simulink model "rti1401_program_controls_2018_test"  (R2017b)
settings: Solver=ode1  StartTime=0.0  StopTime=Inf  FixedStep=0.001  RelTol=1e-3  EnableMultiTasking=on
PreLoadFcn:
  | dataCar
  | load_vars
  | structAero
  | structEstimPar
  | structSensors
  | structSettings
PostLoadFcn:
  | , if any(exist('dsrtsu_mdlpostloadfcn', 'file') == [2, 3, 6]), try dsrtsu_mdlpostloadfcn('Execute', bdroot); catch fprintf('Error in PostLoadFcn (dsrtsu_mdlpostloadfcn) for model "%s":\n %s\n', bdroot, lasterr); end, end,
InitFcn:
  | dataCar
  | load_vars
  | structAero
  | structEstimPar
  | structSensors
  | structSettings
StartFcn:
  | dataCar
  | load_vars
  | structAero
  | structEstimPar
  | structSensors
  | structSettings
values from neighbouring files (symbols this model uses):
  Throttle_limits = [0.15, 0.90, 0.16, 0.92]    [load_vars.m]
undefined symbols (not defined in the file or in its folder): car, sensors
libraries: rtican x44, hdlsllib x32, simulink x8, rti1401lib_II_base x1
(part 1 of 11)
settings Model: DSRTSU_INTERNAL_RTI_VER=490  DSRTSU_INTERNAL_RTI_TYPE=rti1401  DSRTSU_INTERNAL_RTIFPGA=80  DSRTSU_INTERNAL_MDBS_VER=10  Creator=Arthur Coppieters  LastModifiedBy=User
settings OptimizationCC: BlockReduction=off  OptimizeBlockIOStorage=off  BufferReuse=off  GlobalBufferReuse=off  ExpressionFolding=off  LocalBlockOutputs=off  LifeSpan=inf
settings DebuggingCC: SFUnexpectedBacktrackingDiag=warning  SFNoUnconditionalDefaultTransitionDiag=warning  SFExecutionAtInitializationDiag=none
settings HardwareCC: ProdBitPerPointer=32  ProdBitPerSizeT=32  ProdBitPerPtrDiffT=32  ProdLargestAtomicInteger=Integer  ProdEndianess=BigEndian  ProdWordSize=32  ProdHWDeviceType=Custom Processor->Custom  TargetIntDivRoundTo=Zero  TargetEndianess=BigEndian  TargetHWDeviceType=Custom Processor->Custom
settings RTWCC: SystemTargetFile=rti1401.tlc  MakeCommand=make_rti  TemplateMakefile=rti1401.tmf  Description=dSPACE DS1401 Hardware Platform
settings CodeAppCC: StateflowObjectComments=on
settings STFCustomTargetCC: ParMdlRefBuildCompliant=on  GRTInterface=off  SystemTargetFile=rti1401.tlc
settings GRTTargetCC: TargetLangStandard=C89/C90 (ANSI)  CompOptLevelCompliant=off  ConcurrentExecutionCompliant=off  CombineOutputUpdateFcns=off  MatFileLogging=off  CPPClassGenCompliant=off  UseToolchainInfoCompliant=off
settings ConfigComp: CovMetricSettings=dw  CovHtmlReporting=on  CovSaveCumulativeToWorkspaceVar=on  CovSaveSingleToWorkspaceVar=on  CovExternalEMLEnable=off

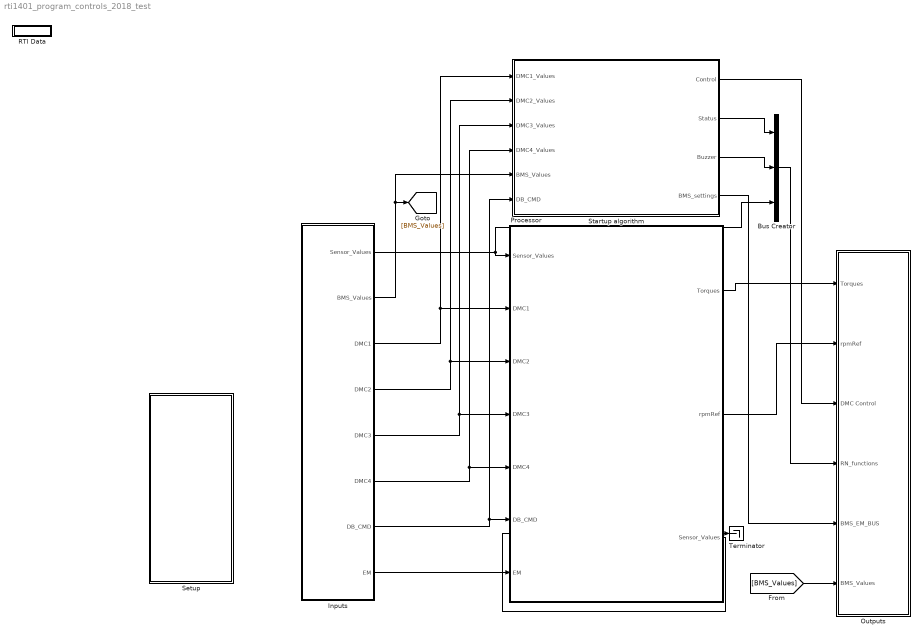
== system rti1401_program_controls_2018_test ==
  Bus Creator : BusCreator  Inputs=3
  Inputs : Subsystem
  Outputs : Subsystem
  Processor : Subsystem
  RTI Data : Subsystem  Tag=struct('RTIDataServer',struct('RTIDataServerVs','2','RTIModelDescription','struct(''main'',''rti1401_program_nova'',''sub'','''',''isMp'',0)'))  LoadFcn="if exist('rtidc'), try,  rtidc('DataHostBlockClbLoad', gcbh); catch, disp(['Warning: ''LoadFcn'' for RTI Data block failed: ' lasterr]); end, end,"  mask(RTI_DATA_HOST){}
      mask help:
      | RTI Data Block.
      | This block is used by RTI to store internal model-dependent data.
      | Please keep this block on the root level of the model. Deleting this block will result in data loss.
      |
      | NEVER DELETE OR COPY THIS BLOCK!
      settings: CopyFcn="if exist('rtidc'), try,  rtidc('DataHostBlockClbCopy', gcbh); catch, disp(['Warning: ''CopyFcn'' for RTI Data block failed: ' lasterr]); end, end,"  DeleteFcn="if exist('rtidc'), try,  rtidc('DataHostBlockClbDelete', gcbh); catch, disp(['Warning: ''DeleteFcn'' for RTI Data block failed: ' lasterr]); end, end,"  ModelCloseFcn="if exist('rtidc'), try,  rtidc('DataHostBlockClbModelClose', gcbh); catch, disp(['Warning: ''ModelCloseFcn'' for RTI Data block failed: ' lasterr]); end, end,"  PreSaveFcn="if exist('rtidc'), try,  rtidc('DataHostBlockClbPreSave', gcbh); catch, disp(['Warning: ''PreSaveFcn'' for RTI Data block failed: ' lasterr]); end, end,"  PostSaveFcn="if exist('rtidc'), try,  rtidc('DataHostBlockClbPostSave', gcbh); catch, disp(['Warning: ''PostSaveFcn'' for RTI Data block failed: ' lasterr]); end, end,"  NameChangeFcn="if exist('rtidc'), try,  rtidc('DataHostBlockClbNameChange', gcbh); catch, disp(['Warning: ''NameChangeFcn'' for RTI Data block failed: ' lasterr]); end, end,"
      mask Help:
      | RTI Data Block.
      | This block is used by RTI to store internal model-dependent data.
      | Please keep this block on the root level of the model. Deleting this block will result in data loss.
      | 
      | NEVER DELETE OR COPY THIS BLOCK!
      mask Display:
      | text(0.5, 0.5, 'RTI Data', 'HorizontalAlignment', 'center');
      | plot([1 0]);
  Setup : Subsystem
  Startup algorithm : Subsystem
  Terminator : Terminator
  wires:
  Inputs/1(Sensor_Values) -> Bus Creator/3, Processor/1("Sensor_Values ")
  Inputs/2(BMS_Values) -> [BMS_Values], Startup algorithm/5(BMS_Values)
  Inputs/3(DMC1) -> Startup algorithm/1(DMC1_Values), Processor/2(DMC1)
  Inputs/4(DMC2) -> Startup algorithm/2(DMC2_Values), Processor/3(DMC2)
  Inputs/5(DMC3) -> Startup algorithm/3(DMC3_Values), Processor/4(DMC3)
  Inputs/6(DMC4) -> Startup algorithm/4(DMC4_Values), Processor/5(DMC4)
  Inputs/7(DB_CMD) -> Startup algorithm/6(DB_CMD), Processor/6(DB_CMD)
  Processor/1(Torques) -> Outputs/1(Torques)
  Processor/2(rpmRef) -> Outputs/2(rpmRef)
  Inputs/8(EM) -> Processor/7(EM)
  Startup algorithm/1(Control) -> Outputs/3(DMC Control)
  Startup algorithm/3(Buzzer) -> Bus Creator/2
  Startup algorithm/2(Status) -> Bus Creator/1
  Bus Creator/1 -> Outputs/4(RN_functions)
  Startup algorithm/4(BMS_settings) -> Outputs/5(BMS_EM_BUS)
  Processor/3(Sensor_Values) -> Terminator/1
  [BMS_Values] -> Outputs/6(BMS_Values)

== system rti1401_program_controls_2018_test/Inputs ==
  Batpack : Subsystem
  Bus Creator : BusCreator  Inputs=4
  Commands : Subsystem
  Drives : Subsystem
  EnergyMeter : Subsystem
  Preprocessor : Subsystem
  Sensors : Subsystem
  Sensor_Values : Outport
  BMS_Values : Outport  Port=2
  DMC1 : Outport  Port=3
  DMC2 : Outport  Port=4
  DMC3 : Outport  Port=5
  DMC4 : Outport  Port=6
  DB_CMD : Outport  Port=7
  EM : Outport  Port=8
  wires:
  Batpack/1(BMS_Values) -> BMS_Values/1
  Drives/1(DMC1) -> DMC1/1
  Drives/2(DMC2) -> DMC2/1
  Drives/3(DMC3) -> DMC3/1
  Drives/4(DMC4) -> DMC4/1
  Commands/1(Dash_Commands) -> DB_CMD/1
  Sensors/1(Front_Sensors) -> Preprocessor/1(Front)
  Sensors/4(Temp_Sensors_Rear) -> Bus Creator/4
  Bus Creator/1 -> Sensor_Values/1  "Sensor_Values"
  Preprocessor/1(Front_proc) -> Bus Creator/1  "Front_proc"
  Sensors/2(Rear_Sensors) -> Preprocessor/2(Rear)
  Preprocessor/2(YRS) -> Bus Creator/2
  Sensors/3(Temp_Sensors_Front) -> Bus Creator/3
  EnergyMeter/1("EM ") -> EM/1

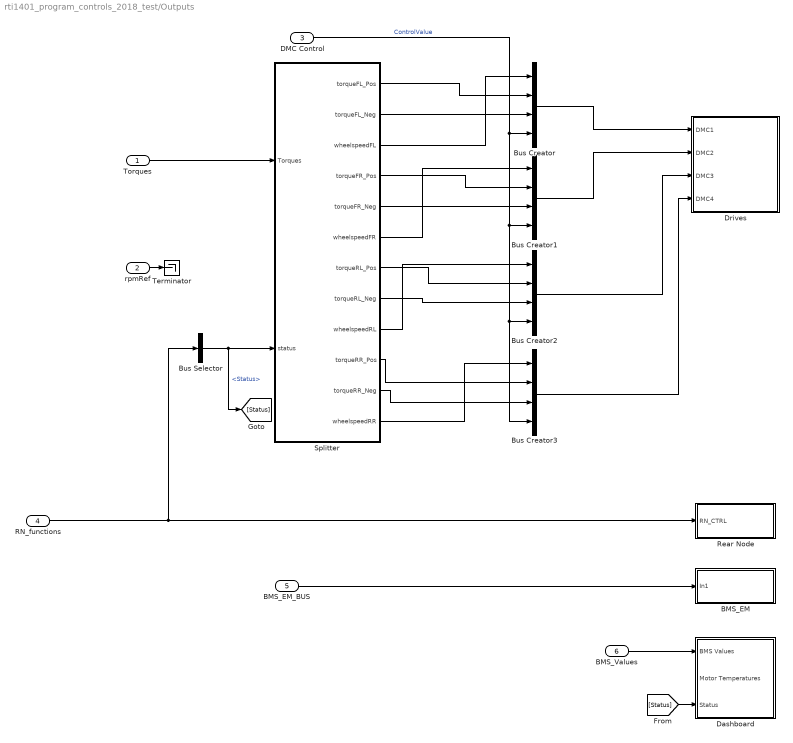
== system rti1401_program_controls_2018_test/Outputs ==
  Torques : Inport
  rpmRef : Inport  Port=2
  DMC Control : Inport  Port=3
  RN_functions : Inport  Port=4
  BMS_EM_BUS : Inport  Port=5
  BMS_Values : Inport  Port=6
  BMS_EM : Subsystem
  Bus Creator{,1..3} (4 alike) : BusCreator  Inputs=4
  Bus Selector : BusSelector  OutputSignals=Status
  Dashboard : Subsystem
  Drives : Subsystem
  Rear Node : Subsystem
  Splitter : MATLAB Function  TreatAsAtomicUnit=on
  Terminator : Terminator
  wires:
  Bus Creator/1 -> Drives/1(DMC1)
  Bus Creator1/1 -> Drives/2(DMC2)
  Bus Creator2/1 -> Drives/3(DMC3)
  Bus Creator3/1 -> Drives/4(DMC4)
  Torques/1 -> Splitter/1(Torques)
  Splitter/1(torqueFL_Pos) -> Bus Creator/2
  Splitter/2(torqueFL_Neg) -> Bus Creator/3
  Splitter/4(torqueFR_Pos) -> Bus Creator1/2
  Splitter/5(torqueFR_Neg) -> Bus Creator1/3
  Splitter/7(torqueRL_Pos) -> Bus Creator2/2
  Splitter/8(torqueRL_Neg) -> Bus Creator2/3
  Splitter/10(torqueRR_Pos) -> Bus Creator3/2
  Splitter/11(torqueRR_Neg) -> Bus Creator3/3
  Splitter/3(wheelspeedFL) -> Bus Creator/1
  Splitter/6(wheelspeedFR) -> Bus Creator1/1
  Splitter/9(wheelspeedRL) -> Bus Creator2/1
  Splitter/12(wheelspeedRR) -> Bus Creator3/1
  BMS_EM_BUS/1 -> BMS_EM/1(In1)
  DMC Control/1 -> Bus Creator3/4, Bus Creator2/4, Bus Creator1/4, Bus Creator/4  "ControlValue"
  RN_functions/1 -> Bus Selector/1, Rear Node/1(RN_CTRL)
  Bus Selector/1 -> [Status], Splitter/2(status)  "<Status>"
  rpmRef/1 -> Terminator/1
  BMS_Values/1 -> Dashboard/1(BMS Values)
  [Status] -> Dashboard/3(Status)

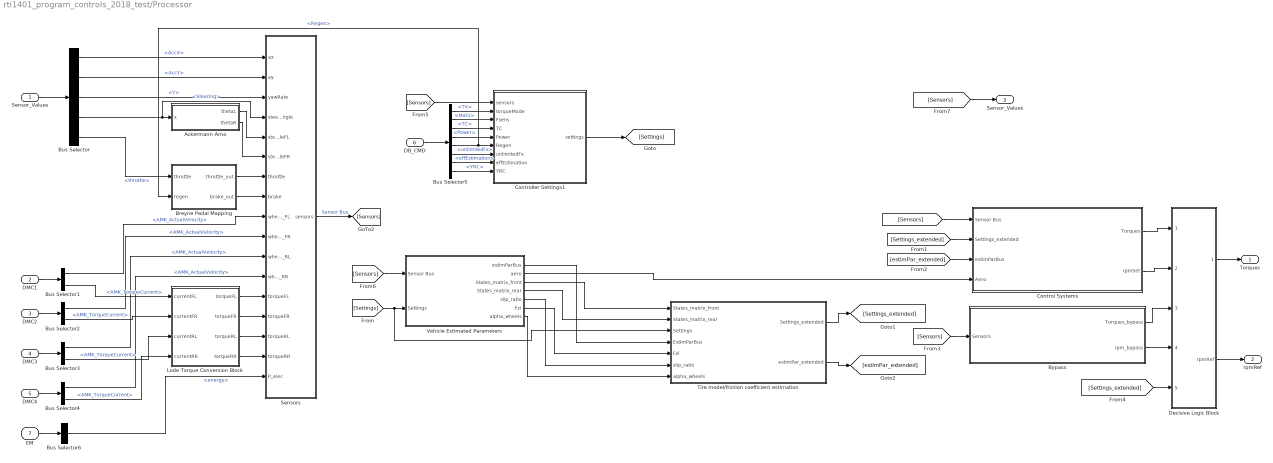
== system rti1401_program_controls_2018_test/Processor ==
  "Sensor_Values " : Inport
  DMC1 : Inport  Port=2
  DMC2 : Inport  Port=3
  DMC3 : Inport  Port=4
  DMC4 : Inport  Port=5
  DB_CMD : Inport  Port=6
  EM : Inport  Port=7
  Ackermann Arno : MATLAB Function  TreatAsAtomicUnit=on
  Breyne Pedal Mapping : MATLAB Function  TreatAsAtomicUnit=on
  Bus Selector : BusSelector  OutputSignals=signal2.AccX,signal2.AccY,signal2.Y,Front_proc.Steering,Front_proc.throttle
  Bus Selector{1..4} (4 alike) : BusSelector  OutputSignals=AMK_ActualVelocity,AMK_TorqueCurrent
  Bus Selector5 : BusSelector  OutputSignals=TV,MxFz,TC,Power,Regen,unlimitedFx,effEstimation,YRC
  Bus Selector6 : BusSelector  OutputSignals=energy
  Bypass : Subsystem
  Control Systems : Subsystem
  Controller Settings1 : MATLAB Function  TreatAsAtomicUnit=on
  Decisive Logic Block : Subsystem
  Lode Torque Conversion Block : MATLAB Function  TreatAsAtomicUnit=on
  Sensors : MATLAB Function  TreatAsAtomicUnit=on
  Tire model/friction coefficient estimation : Subsystem
  Vehicle Estimated Parameters : Subsystem
  Torques : Outport
  rpmRef : Outport  Port=2
  Sensor_Values : Outport  Port=3
  wires:
  Controller Settings1/1(settings) -> [Settings]
  [Settings_extended] -> Control Systems/2(Settings_extended)
  Control Systems/1(Torques) -> Decisive Logic Block/1(TorqueController)
  Decisive Logic Block/1(Torques) -> Torques/1
  [Settings_extended] -> Decisive Logic Block/5(Settings)
  Control Systems/2(rpmSet) -> Decisive Logic Block/2(rpmController)
  DB_CMD/1 -> Bus Selector5/1
  Decisive Logic Block/2(rpmRef) -> rpmRef/1
  [Sensors] -> Vehicle Estimated Parameters/1(Sensor Bus)
  [Sensors] -> Control Systems/1(Sensor Bus)
  [Sensors] -> Sensor_Values/1
  [Sensors] -> Controller Settings1/1(sensors)
  Bus Selector5/8 -> Controller Settings1/9(YRC)  "<YRC>"
  Bus Selector5/7 -> Controller Settings1/8(effEstimation)  "<effEstimation>"
  Bus Selector5/6 -> Controller Settings1/7(unlimitedFx)  "<unlimitedFx>"
  Bus Selector5/5 -> Breyne Pedal Mapping/2(regen), Controller Settings1/6(Regen)  "<Regen>"
  Bus Selector5/4 -> Controller Settings1/5(Power)  "<Power>"
  Bus Selector5/3 -> Controller Settings1/4(TC)  "<TC>"
  Bus Selector5/2 -> Controller Settings1/3(Fsens)  "<MxFz>"
  Bus Selector5/1 -> Controller Settings1/2(torqueMode)  "<TV>"
  Bypass/1(Torques_bypass) -> Decisive Logic Block/3(TorqueBypass)
  Bypass/2(rpm_bypass) -> Decisive Logic Block/4(rpmBypass)
  [Sensors] -> Bypass/1(Sensors)
  "Sensor_Values "/1 -> Bus Selector/1
  DMC1/1 -> Bus Selector1/1
  DMC2/1 -> Bus Selector2/1
  DMC3/1 -> Bus Selector3/1
  DMC4/1 -> Bus Selector4/1
  Bus Selector/4 -> Sensors/4(steeringAngle), Ackermann Arno/1(x)  "<Steering>"
  Bus Selector/3 -> Sensors/3(yawRate)  "<Y>"
  Bus Selector/2 -> Sensors/2(ay)  "<AccY>"
  Bus Selector/1 -> Sensors/1(ax)  "<AccX>"
  Bus Selector1/1 -> Sensors/9(wheelspeed_FL)  "<AMK_ActualVelocity>"
  Bus Selector1/2 -> Lode Torque Conversion Block/1(currentFL)  "<AMK_TorqueCurrent>"
  Bus Selector2/1 -> Sensors/10(wheelspeed_FR)  "<AMK_ActualVelocity>"
  Bus Selector2/2 -> Lode Torque Conversion Block/2(currentFR)  "<AMK_TorqueCurrent>"
  Bus Selector3/1 -> Sensors/11(wheelspeed_RL)  "<AMK_ActualVelocity>"
  Bus Selector3/2 -> Lode Torque Conversion Block/3(currentRL)  "<AMK_TorqueCurrent>"
  Bus Selector4/1 -> Sensors/12(wheelspeed_RR)  "<AMK_ActualVelocity>"
  Bus Selector4/2 -> Lode Torque Conversion Block/4(currentRR)  "<AMK_TorqueCurrent>"
  Ackermann Arno/1(thetaL) -> Sensors/5(steerAngleFL)
  Ackermann Arno/2(thetaR) -> Sensors/6(steerAngleFR)
  Sensors/1(sensors) -> [Sensors]  "Sensor Bus"
  EM/1 -> Bus Selector6/1
  Bus Selector6/1 -> Sensors/17(P_elec)  "<energy>"
  Lode Torque Conversion Block/4(torqueRR) -> Sensors/16(torqueRR)
  Lode Torque Conversion Block/1(torqueFL) -> Sensors/13(torqueFL)
  Lode Torque Conversion Block/2(torqueFR) -> Sensors/14(torqueFR)
  Lode Torque Conversion Block/3(torqueRL) -> Sensors/15(torqueRL)
  Breyne Pedal Mapping/2(brake_out) -> Sensors/8(brake)
  Breyne Pedal Mapping/1(throttle_out) -> Sensors/7(throttle)
  Bus Selector/5 -> Breyne Pedal Mapping/1(throttle)  "<throttle>"
  Vehicle Estimated Parameters/2(aero) -> Control Systems/4(Aero)
  Vehicle Estimated Parameters/1(estimParBus) -> Tire model/friction coefficient estimation/4(EstimParBus)
  [Settings] -> Tire model/friction coefficient estimation/3(Settings), Vehicle Estimated Parameters/2(Settings)
  Vehicle Estimated Parameters/3(States_matrix_front) -> Tire model/friction coefficient estimation/1(States_matrix_front)
  Vehicle Estimated Parameters/4(States_matrix_rear) -> Tire model/friction coefficient estimation/2(States_matrix_rear)
  Vehicle Estimated Parameters/5(slip_ratio) -> Tire model/friction coefficient estimation/6(slip_ratio)
  Tire model/friction coefficient estimation/1(Settings_extended) -> [Settings_extended]
  Tire model/friction coefficient estimation/2(estimPar_extended) -> [estimPar_extended]
  [estimPar_extended] -> Control Systems/3(estimParBus)
  Vehicle Estimated Parameters/6(Fzi) -> Tire model/friction coefficient estimation/5(Fzi)
  Vehicle Estimated Parameters/7(alpha_wheels) -> Tire model/friction coefficient estimation/7(alpha_wheels)

== system rti1401_program_controls_2018_test/RTI Data ==
  RTI Data Store : Subsystem  Tag="struct('private',struct('version',struct('dsVer',uint32(2),'dsVerCreation',uint32(2),'RTI',struct('ver','7.7','type','RTI1401')),'access',struct('type','Model','isPerm',1,'created',['26-Jun-2017 18:43:42'],'modified',['12-Jul-2017 12:28:20'],'location','')),'public',struct('main',struct('data',[]),'sub',struct('name',{{'rti1401_program_nova'}},'data',{{struct('TH',struct('thTaskInfo',struct('taskType',{'TIMER','HWINT','TMRINT','SWINT','GLINT'},'tasksNumOf',{3,0,0,0,0},'srcIds',{{'TIMERA','TIMERA2','TIMERA3'},{},{},{},{}},'taskNames',{{['Timer Task 1'],['Timer Task 2'],['Timer Task 3']},{},{},{},{}})),'th_tc',struct('dataType',{'TASK','TASK','TASK'},'taskGroupId',{'','',''},'taskGroupList',{{},{},{}},'taskSchedulingPolicy',{'FCFS','FCFS','FCFS'},'taskType',{'TIMER','TIMER','TIMER'},'blkh',{-1,-1,-1},'srcId',{'TIMERA','TIMERA2','TIMERA3'},'srcSgnName',{['Timer A interrupt'],['Timer Task 1'],['Timer Task 1']},'srcCpuName',{'','',''},'taskName',{['Timer Task 1  [0.001] s'],['Timer Task 2  [0.01] s'],['Timer Task 3  [0.02] s']},'taskNameDisplayExt',{'','',''},'smplTime',{0.001,0.01,0.02},'smplTimeOffs',{0,0,0},'hasFixedPriority',{0,0,0},'priority',{1,2,3},'hasFixedOvc',{0,0,0},'ovcType',{1,1,1},'ovcMax',{1,1,1}),'tc_th',struct('dataType',{'TASK','TASK','TASK'},'taskGroupId',{'','',''},'taskGroupList',{{},{},{}},'taskSchedulingPolicy',{'FCFS','FCFS','FCFS'},'taskType',{'TIMER','TIMER','TIMER'},'blkh',{-1,-1,-1},'srcId',{'TIMERA','TIMERA2','TIMERA3'},'srcSgnName',{['Timer A interrupt'],['Timer Task 1'],['Timer Task 1']},'srcCpuName',{'','',''},'taskName',{['Timer Task 1  [0.001] s'],['Timer Task 2  [0.01] s'],['Timer Task 3  [0.02] s']},'taskNameDisplayExt',{'','',''},'smplTime',{0.001,0.01,0.02},'smplTimeOffs',{0,0,0},'hasFixedPriority',{0,0,0},'priority',{1,2,3},'hasFixedOvc',{0,0,0},'ovcType',{1,1,1},'ovcMax',{1,1,1}))}})))"  mask(RTI_DATA_STORE){}
      mask help:
      | RTI Data Store Block. This block is used by RTI to store internal model dependent data. Deleting this block will result in data loss.
      |
      | NEVER DELETE, COPY, OR MODIFY THIS BLOCK!
      mask Help:
      | RTI Data Store Block. This block is used by RTI to store internal model dependent data. Deleting this block will result in data loss.
      | 
      | NEVER DELETE, COPY, OR MODIFY THIS BLOCK!
      mask Display: text(0.5, 0.5, ' ', 'HorizontalAlignment', 'center');
